simulink model "Bai03"  (R2019a)
settings: Solver=VariableStepAuto  StartTime=0.0  StopTime=10.0  RelTol=1e-3
settings Model: Creator=ASUS  LastModifiedBy=ASUS

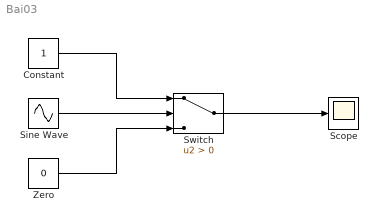
== system Bai03 ==
  Constant : Constant
  Scope : Scope
  Sine Wave : Sin  SampleTime=0
  Switch : Switch  Criteria=u2 > Threshold
  Zero : Constant  Value=0  OutDataTypeStr=Inherit: Inherit via back propagation
  wires:
  Constant/1 -> Switch/1
  Zero/1 -> Switch/3
  Switch/1 -> Scope/1
  Sine Wave/1 -> Switch/2
